simulink subsystem "Vehicle_Model_Simplified"  (R2023b)
settings: Solver=VariableStepAuto  StartTime=0.0  StopTime=10.0  RelTol=1e-3
undefined symbols (not defined in the file): chassis, dZ, F0z, fractalcoef, IMU_accel, IMU_gyro, IMU_mag, phi, powertrain, psi, sim, suspension, theta, VEH, X, Xdot, Y, Ydot, Z, Zdot
libraries: vehdynlibtire x10, vehdynlibsuspension x8, autolibutils x5, sharedtransform x5, shared6dof x2, sensorgpslib x1, mspsensorlib x1, dspstat3 x1, vehdynlibeom x1, vehdynlibtirecommon x1
(part 1 of 6)
settings Model: Creator=Inver  LastModifiedBy=Inver
settings OptimizationCC: ReuseModelBlockBuffer=off

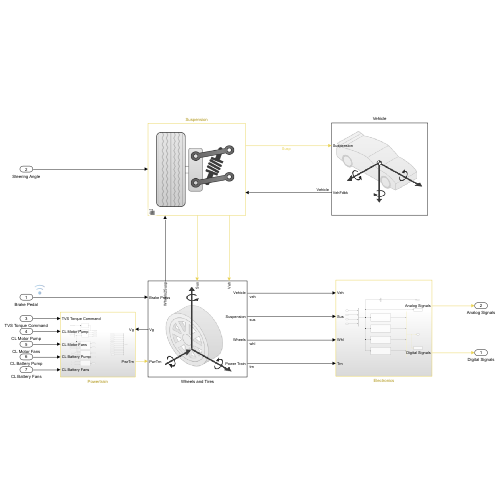
[thumbnail: Simulink's stored preview of the top-level diagram]
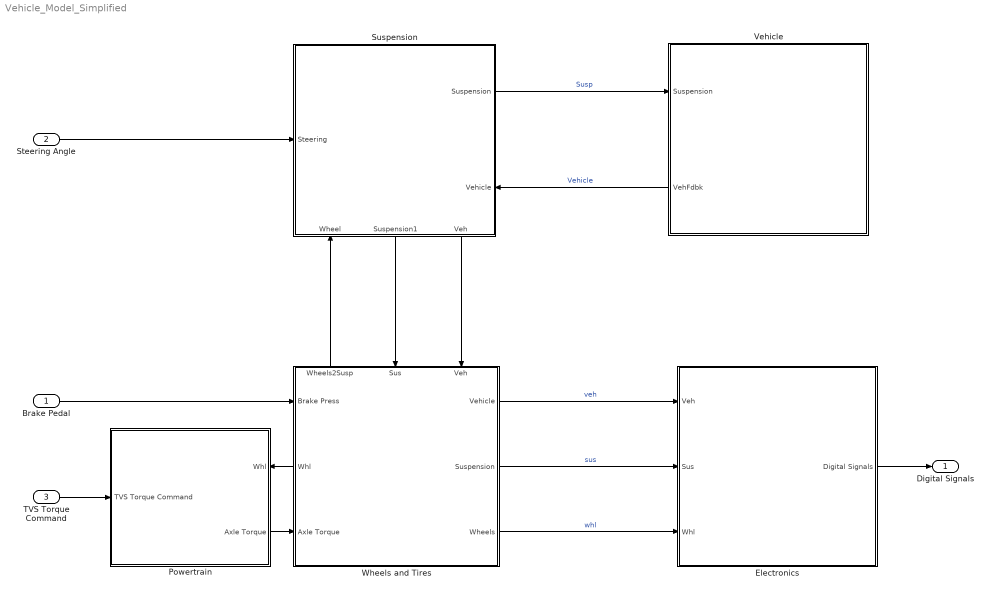
== system Vehicle_Model_Simplified ==
  Brake Pedal : Inport
  Steering Angle : Inport  Port=2
  TVS Torque Command : Inport  Port=3
  Electronics : Subsystem
  Powertrain : Subsystem
      settings: PortSchema="{\"entries\":[{\"content\":{\"sides\":[{\"content\":{\"connectorIds\":[\"In1\"]},\"type\":\"ConnectorPlacement.EquallySpacedRectSide\",\"uuid\":\"0d21e996-4b5b-4450-af88-3d06a2954fb0\"},{\"content\":{\"connectorIds\":[\"In2\",\"Out1\"],\"side\":\"RIGHT\"},\"type\":\"ConnectorPlacement.EquallySpacedRectSide\",\"uuid\":\"9f5ebd0c-1dcb-4dff-b45c-eedc8c3fdf23\"},{\"content\":{\"side\":\"TOP\"},\"type\":\"ConnectorPlacement.EquallySpacedRectSide\",\"uuid\":\"a4defc37-f0d5-4878-ad0c-0744c40eb739\"}]},\"type\":\"ConnectorPlacement.EquallySpacedConnector\",\"uuid\":\"e0fe36d7-0668-4ee0-8075-231a8c6bd792\"}],\"packageUris\":[\"http://schema.mathworks.com/mf0/Connector/R2020b\"],\"version\":\"1.0\"}"
  Suspension : Subsystem  Variant=on  VariantControlMode=label  LabelModeActiveChoice=1
      settings: PortSchema="{\"entries\":[{\"content\":{\"sides\":[{\"content\":{\"connectorIds\":[\"In1\"]},\"type\":\"ConnectorPlacement.EquallySpacedRectSide\",\"uuid\":\"d90bf910-501d-4dd1-a367-d76bd42ab174\"},{\"content\":{\"connectorIds\":[\"Out1\",\"In3\"],\"side\":\"RIGHT\"},\"type\":\"ConnectorPlacement.EquallySpacedRectSide\",\"uuid\":\"1fe7da07-1086-4d5e-8baf-d5d069455d6e\"},{\"content\":{\"connectorIds\":[],\"side\":\"TOP\"},\"type\":\"ConnectorPlacement.EquallySpacedRectSide\",\"uuid\":\"6ff63b9e-45bb-47e9-90cd-47f8e0815e57\"},{\"content\":{\"connectorIds\":[\"In2\",\"Out2\",\"Out3\"],\"side\":\"BOTTOM\"},\"type\":\"ConnectorPlacement.EquallySpacedRectSide\",\"uuid\":\"116c6de0-7bfa-4dc1-bfd0-57a2fffb3aa0\"}]},\"type\":\"ConnectorPlacement.EquallySpacedConnector\",\"uuid\":\"6475b998-12b0-4b0e-8a20-c379b8e08c7c\"}],\"packageUris\":[\"http://schema.mathworks.com/mf0/Connector/R2020b\"],\"version\":\"1.0\"}"
      mask Display:
      | switch str2num(get_param(gcb,'ActiveVariant'))
      |     case 1
      |         image('suspdw.png');
      |     case 2
      |         image([imread('suspindmap.png');imread('suspsamap.png')]);
      |     case 3
      |          image([imread('suspmacp.png');imread('suspsacoil.png')]);
      |     case 4
      |          image('suspmacp.png');
      |     case 5
      |          image('suspindmap.png');
      |     case 6
      |          image('suspkandc.png');
      | end
  Vehicle : Subsystem
      settings: PortSchema="{\"entries\":[{\"content\":{\"sides\":[{\"content\":{\"connectorIds\":[\"In1\",\"Out1\"]},\"type\":\"ConnectorPlacement.EquallySpacedRectSide\",\"uuid\":\"63fa377f-0583-4c60-bac7-9bd73dadd9a1\"},{\"content\":{\"connectorIds\":[],\"side\":\"RIGHT\"},\"type\":\"ConnectorPlacement.EquallySpacedRectSide\",\"uuid\":\"7f668e34-aa5e-4f2f-9be8-80fbb83ff2c8\"},{\"content\":{\"connectorIds\":[],\"side\":\"TOP\"},\"type\":\"ConnectorPlacement.EquallySpacedRectSide\",\"uuid\":\"511f439c-568f-45f1-9ff4-54e644eb8180\"}]},\"type\":\"ConnectorPlacement.EquallySpacedConnector\",\"uuid\":\"b54bf87e-fa06-468b-8fa9-38148d60ed3d\"}],\"packageUris\":[\"http://schema.mathworks.com/mf0/Connector/R2020b\"],\"version\":\"1.0\"}"
      mask Display: image('6dofcar.png');
  Wheels and Tires : Subsystem
      settings: PortSchema="{\"entries\":[{\"content\":{\"sides\":[{\"content\":{\"connectorIds\":[\"In1\",\"Out5\",\"In2\"]},\"type\":\"ConnectorPlacement.EquallySpacedRectSide\",\"uuid\":\"77263124-783e-4307-b979-a6212540af24\"},{\"content\":{\"connectorIds\":[\"Out1\",\"Out2\",\"Out3\"],\"side\":\"RIGHT\"},\"type\":\"ConnectorPlacement.EquallySpacedRectSide\",\"uuid\":\"cb03b446-69c2-4dbf-929b-d33818acfe8b\"},{\"content\":{\"connectorIds\":[\"Out4\",\"In3\",\"In4\"],\"side\":\"TOP\"},\"type\":\"ConnectorPlacement.EquallySpacedRectSide\",\"uuid\":\"8e7e4023-62e5-48a8-8666-b4c8bb14cd01\"}]},\"type\":\"ConnectorPlacement.EquallySpacedConnector\",\"uuid\":\"1061f0db-ec8e-49bd-8d66-b4a53eaeacfa\"}],\"packageUris\":[\"http://schema.mathworks.com/mf0/Connector/R2020b\"],\"version\":\"1.0\"}"
      mask Display: image('wheel3dof.png')
  Digital Signals : Outport  PortDimensions={292}
  wires:
  Wheels and Tires/1(Vehicle) -> Electronics/1(Veh)  "veh"
  Electronics/1(Digital Signals) -> Digital Signals/1
  Vehicle/1(VehFdbk) -> Suspension/3(Vehicle)  "Vehicle"
  Suspension/2(Suspension1) -> Wheels and Tires/3(Sus)
  TVS Torque Command/1 -> Powertrain/1(TVS Torque Command)
  Steering Angle/1 -> Suspension/1(Steering)
  Wheels and Tires/4(Wheels2Susp) -> Suspension/2(Wheel)
  Brake Pedal/1 -> Wheels and Tires/1(Brake Press)
  Wheels and Tires/2(Suspension) -> Electronics/2(Sus)  "sus"
  Suspension/1(Suspension) -> Vehicle/1(Suspension)  "Susp"
  Suspension/3(Veh) -> Wheels and Tires/4(Veh)
  Powertrain/1(Axle Torque) -> Wheels and Tires/2(Axle Torque)
  Wheels and Tires/3(Wheels) -> Electronics/3(Whl)  "whl"
  Wheels and Tires/5(Whl) -> Powertrain/2(Whl)

== system Vehicle_Model_Simplified/Electronics ==
  Veh : Inport
  Sus : Inport  Port=2
  Whl : Inport  Port=3
  All Veh Info : BusCreator  Inputs=3
  Corner Dynamics Sensors : Subsystem
  Digital SIgnals : BusCreator  Inputs=2
  Navigation Sensors : Subsystem
  To Workspace : ToWorkspace  VariableName=Digital_Signals  SaveFormat=Timeseries  SampleTime=-1
  To Workspace1 : ToWorkspace  VariableName=Vehicle_Signals  SaveFormat=Timeseries  SampleTime=-1
  Digital Signals : Outport
  wires:
  Sus/1 -> All Veh Info/2
  Whl/1 -> All Veh Info/3
  Navigation Sensors/1(Navigation Sensors) -> Digital SIgnals/1  "Navigation Sensors"
  Corner Dynamics Sensors/1(Corner Dynamics Sensors) -> Digital SIgnals/2  "Corner Dynamics Sensors"
  Digital SIgnals/1 -> Digital Signals/1, To Workspace/1  "Digital Signls"
  All Veh Info/1 -> To Workspace1/1, Navigation Sensors/1(Analog Signals), Corner Dynamics Sensors/1(Analog Signals)
  Veh/1 -> All Veh Info/1  "veh"

== system Vehicle_Model_Simplified/Powertrain ==
  TVS Torque Command : Inport
  Whl : Inport  Port=2
  Bus Selector : BusSelector  OutputSignals=TireFrame.Omega
  Drivetrain : Subsystem
  Gain : Gain  Gain=sim.top_parameters.MOTOR_ENABLE
  Gain1 : Gain  Gain=powertrain.gearbox.gr
  HV Battery : Subsystem
  Axle Torque : Outport
  wires:
  Gain1/1 -> Drivetrain/3(motor speed)
  Whl/1 -> Bus Selector/1
  Drivetrain/3(wheel torque) -> Axle Torque/1
  Bus Selector/1 -> Gain1/1  "<Omega>"
  TVS Torque Command/1 -> Drivetrain/2(throttle)
  HV Battery/1(battery_V) -> [BattV], Gain/1, Drivetrain/1(battery voltage)
  Drivetrain/1(battery current) -> [BattI], HV Battery/1(battery_I)
  Drivetrain/2(motor current) -> [MotI]
  Gain/1 -> [MotV]

== system Vehicle_Model_Simplified/Suspension ==
  Steering : Inport
  Wheel : Inport  Port=2
  Vehicle : Inport  Port=3
  Double Wishbone Suspension : Subsystem  VariantControl=1
      mask Display: image('suspdw.png');
  Independent Mapped Front Suspension Mapped Solid Axle Rear Suspension : Subsystem  VariantControl=2
      mask Display: image([imread('suspindmap.png');imread('suspsamap.png')]);
  Kinematics and Compliance Independent Suspension : Subsystem  VariantControl=6
      mask Display: image('suspkandc.png');
  MacPherson Front Suspension Solid Axle Rear Suspension : Subsystem  VariantControl=3
      mask Display: image([imread('suspmacp.png');imread('suspsacoil.png')]);
  MacPherson Suspension : Subsystem  VariantControl=4
      mask Display: image('suspmacp.png');
  Mapped Suspension : Subsystem  VariantControl=5
      mask Display: image('suspindmap.png');
  Suspension : Outport  VectorParamsAs1DForOutWhenUnconnected=off
  Suspension1 : Outport  Port=2  VectorParamsAs1DForOutWhenUnconnected=off
  Veh : Outport  Port=3  VectorParamsAs1DForOutWhenUnconnected=off

== system Vehicle_Model_Simplified/Vehicle ==
  Suspension : Inport
  6DOF : Subsystem  VariantControl=1
  Constant : Constant  Value=[0 0 0]
  VehFdbk : Outport  VectorParamsAs1DForOutWhenUnconnected=off
  wires:
  6DOF/1(VehFdbk) -> VehFdbk/1  "VehFdbk"
  Constant/1 -> 6DOF/2(Wind)
  Suspension/1 -> 6DOF/1(Suspension)

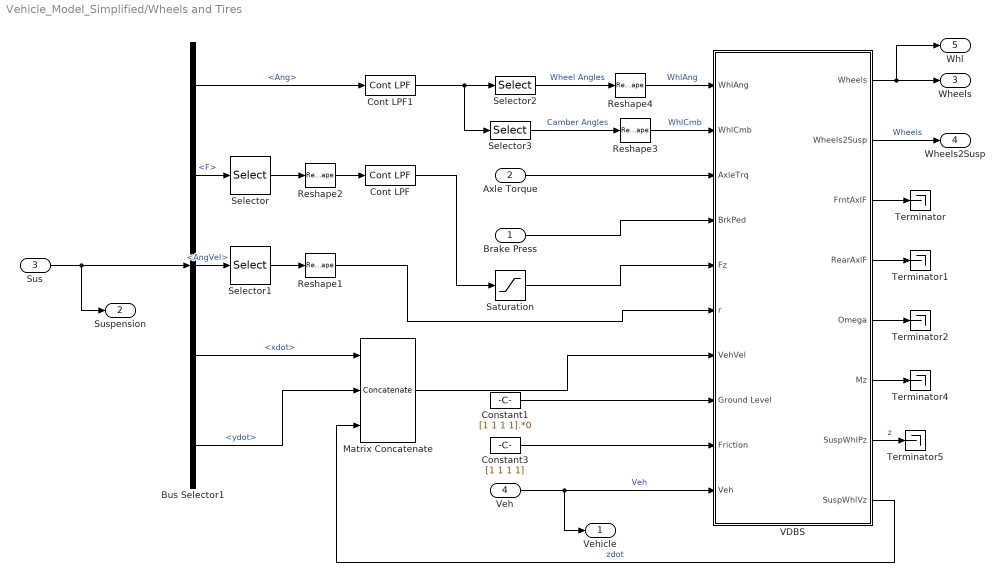
== system Vehicle_Model_Simplified/Wheels and Tires ==
  Brake Press : Inport  Unit=Pa
  Axle Torque : Inport  Port=2
  Sus : Inport  Port=3
  Veh : Inport  Port=4
  Bus Selector1 : BusSelector  OutputSignals=Whl.Ang,Whl.F,Whl.AngVel,Whl.xdot,Whl.ydot
  Constant1 : Constant  Value=[1 1 1 1].*0
  Constant3 : Constant  Value=[1 1 1 1]
  Cont LPF : autolibutils/Cont LPF  wc=100*2*pi  AbsoluteTolerance=auto  aMode=2
  Cont LPF1 : autolibutils/Cont LPF  wc=100*2*pi  AbsoluteTolerance=auto  aMode=2
  Matrix Concatenate : Concatenate  NumInputs=3  Mode=Multidimensional array
  Reshape{1..4} (4 alike) : Reshape
  Saturation : Saturate  UpperLimit=inf  LowerLimit=-10*9.81*2000  ZeroCross=off
  Selector : Selector  NumberOfDimensions=2  InputPortWidth=3  IndexOptions=Index vector (dialog),Select all  Indices=[3],1  OutputSizes=1,1
  Selector1 : Selector  NumberOfDimensions=2  InputPortWidth=1  IndexOptions=Index vector (dialog),Select all  Indices=[3],1  OutputSizes=1,1
  Selector2 : Selector  NumberOfDimensions=2  InputPortWidth=3  IndexOptions=Index vector (dialog),Select all  Indices=3,1  OutputSizes=1,1
  Selector3 : Selector  NumberOfDimensions=2  InputPortWidth=3  IndexOptions=Index vector (dialog),Select all  Indices=1,1  OutputSizes=1,1
  Terminator{,1..2,4..5} (5 alike) : Terminator
  VDBS : Subsystem  VariantControl=0
  Vehicle : Outport  VectorParamsAs1DForOutWhenUnconnected=off
  Suspension : Outport  Port=2  VectorParamsAs1DForOutWhenUnconnected=off
  Wheels : Outport  Port=3  VectorParamsAs1DForOutWhenUnconnected=off
  Wheels2Susp : Outport  Port=4  VectorParamsAs1DForOutWhenUnconnected=off
  Whl : Outport  Port=5  VectorParamsAs1DForOutWhenUnconnected=off
  wires:
  Axle Torque/1 -> VDBS/3(AxleTrq)
  Bus Selector1/2 -> Selector/1  "<F>"
  VDBS/3(FrntAxlF) -> Terminator/1
  VDBS/4(RearAxlF) -> Terminator1/1
  VDBS/6(Mz) -> Terminator4/1
  Selector1/1 -> Reshape1/1
  Matrix Concatenate/1 -> VDBS/7(VehVel)
  Reshape4/1 -> VDBS/1(WhlAng)  "WhlAng"
  Reshape3/1 -> VDBS/2(WhlCmb)  "WhlCmb"
  Selector/1 -> Reshape2/1
  Saturation/1 -> VDBS/5(Fz)
  Constant1/1 -> VDBS/8(Ground Level)
  VDBS/8(SuspWhlVz) -> Matrix Concatenate/3  "zdot"
  Bus Selector1/1 -> Cont LPF1/1  "<Ang>"
  Selector3/1 -> Reshape3/1  "Camber Angles"
  Sus/1 -> Suspension/1, Bus Selector1/1
  Bus Selector1/4 -> Matrix Concatenate/1  "<xdot>"
  Bus Selector1/5 -> Matrix Concatenate/2  "<ydot>"
  VDBS/7(SuspWhlPz) -> Terminator5/1  "z"
  Reshape2/1 -> Cont LPF/1
  Bus Selector1/3 -> Selector1/1  "<AngVel>"
  Reshape1/1 -> VDBS/6(r)
  Brake Press/1 -> VDBS/4(BrkPed)
  Constant3/1 -> VDBS/9(Friction)
  Cont LPF/1 -> Saturation/1
  Cont LPF1/1 -> Selector3/1, Selector2/1
  Selector2/1 -> Reshape4/1  "Wheel Angles"
  Veh/1 -> Vehicle/1, VDBS/10(Veh)  "Veh"
  VDBS/2(Wheels2Susp) -> Wheels2Susp/1  "Wheels"
  VDBS/1(Wheels) -> Wheels/1, Whl/1
  VDBS/5(Omega) -> Terminator2/1

== system Vehicle_Model_Simplified/Electronics/Corner Dynamics Sensors ==
  Analog Signals : Inport
  Bus Creator10 : BusCreator  Inputs=4
  Bus Selector : BusSelector  OutputSignals=whl.TireFrame.Omega,sus.Sus.steering_angle,sus.Sus.shock_length,whl.TireFrame.GndFz
  Delay15 : Delay  InitialCondition=ones(1, 4, 2).*sim.IC.omega_IC
  Delay16 : Delay  InitialCondition=[1 1].*sim.IC.theta_IC
  Delay17 : Delay  InitialCondition=[1 1; 1 1; 1 1; 1 1].*sim.IC.shock_length_IC
  Delay18 : Delay  InitialCondition=[1 1; 1 1; 1 1; 1 1].*sim.IC.Fz_IC
  Saturation15 : Saturate  UpperLimit=sim.range.SHOCK_LENGTH_MAX  LowerLimit=sim.range.SHOCK_LENGTH_MIN
  Saturation16 : Saturate  UpperLimit=sim.range.OMEGA_MAX  LowerLimit=sim.range.OMEGA_MIN
  Saturation17 : Saturate  UpperLimit=sim.range.FZ_MAX  LowerLimit=sim.range.FZ_MIN
  Saturation3 : Saturate  UpperLimit=sim.range.CENTER_STEER_ANGLE_MAX  LowerLimit=-sim.range.CENTER_STEER_ANGLE_MAX
  Transpose : Math  Operator=transpose
  Zero-Order Hold{15..18} (4 alike) : ZeroOrderHold  SampleTime=sim.timing.duplicate
  Corner Dynamics Sensors : Outport
  wires:
  Transpose/1 -> Zero-Order Hold15/1  "omega"
  Bus Selector/1 -> Transpose/1  "<Omega>"
  Zero-Order Hold18/1 -> Delay18/1
  Delay18/1 -> Saturation17/1
  Zero-Order Hold15/1 -> Delay15/1
  Zero-Order Hold16/1 -> Delay16/1
  Saturation17/1 -> Bus Creator10/4  "FZ"
  Saturation3/1 -> Bus Creator10/2  "theta"
  Bus Selector/3 -> Zero-Order Hold17/1  "<shock_length>"
  Saturation15/1 -> Bus Creator10/3  "shock_L"
  Saturation16/1 -> Bus Creator10/1  "omega"
  Bus Selector/4 -> Zero-Order Hold18/1  "<GndFz>"
  Delay16/1 -> Saturation3/1
  Bus Selector/2 -> Zero-Order Hold16/1  "<steering_angle>"
  Delay17/1 -> Saturation15/1
  Delay15/1 -> Saturation16/1
  Zero-Order Hold17/1 -> Delay17/1
  Bus Creator10/1 -> Corner Dynamics Sensors/1
  Analog Signals/1 -> Bus Selector/1

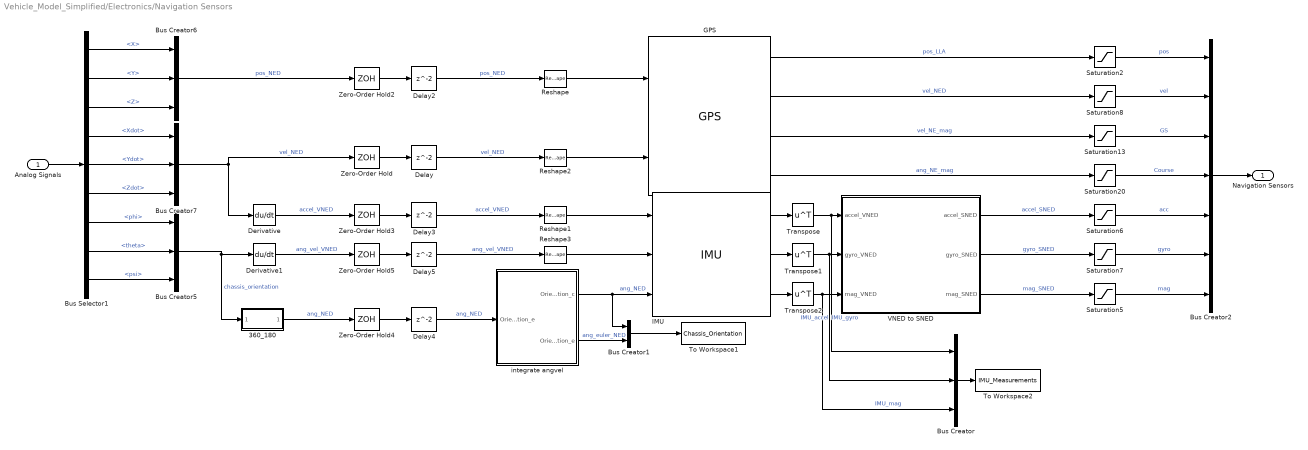
== system Vehicle_Model_Simplified/Electronics/Navigation Sensors ==
  Analog Signals : Inport
  360_180 : Subsystem
  Bus Creator : BusCreator  Inputs=IMU_accel,IMU_gyro,IMU_mag
  Bus Creator1 : BusCreator  Inputs=2
  Bus Creator2 : BusCreator  Inputs=7
  Bus Creator5 : BusCreator  Inputs=phi,theta,psi
  Bus Creator6 : BusCreator  Inputs=X,Y,Z
  Bus Creator7 : BusCreator  Inputs=Xdot,Ydot,Zdot
  Bus Selector1 : BusSelector  OutputSignals=veh.InertFrm.Cg.Disp.X,veh.InertFrm.Cg.Disp.Y,veh.InertFrm.Cg.Disp.Z,veh.InertFrm.Cg.Vel.Xdot,veh.InertFrm.Cg.Vel.Ydot,veh.InertFrm.Cg.Vel.Zdot,veh.InertFrm.Cg.Ang.phi,veh.InertFrm.Cg.Ang.theta,veh.InertFrm.Cg.Ang.psi
  Delay : Delay  InitialCondition=([1;1]*sim.IC.vel_IC)'
  Delay2 : Delay  InitialCondition=[1 1; 1 1; 1 1].*sim.IC.pos_IC
  Delay3 : Delay  InitialCondition=[1 1; 1 1; 1 1].*sim.IC.acc_IC
  Delay4 : Delay  InitialCondition=[1 1; 1 1; 1 1].*sim.IC.ang_IC
  Delay5 : Delay  InitialCondition=[1 1; 1 1; 1 1].*sim.IC.ang_vel_IC
  Derivative : Derivative
  Derivative1 : Derivative
  GPS : sensorgpslib/GPS  DispRefFrame=NED  PositionInputFormat=Local  ReferenceLocation=sim.IC.location_lla_IC  HorizontalPositionAccuracy=sensor.gps.GPS_Z_ACCURACY  VerticalPositionAccuracy=sensor.gps.GPS_XY_ACCURACY  VelocityAccuracy=sensor.gps.GPS_V_ACCURACY  DecayFactor=sensor.gps.GPS_NOISE_FACTOR  SeedDouble=sensor.gps.r_GPS  SimulateUsing=Interpreted execution
      settings: LibrarySourceBlock=mspsensorlib/GPS
  IMU : mspsensorlib/IMU  DispRefFrame=NED  TemperaturePort=off  Temperature=25  MagneticFieldPort=off  MagneticFieldNED=sim.IC.mag_field_IC  MagneticFieldENU=[ -2.4169, 27.5550, 16.0849 ]  SeedDouble=sensor.imu.r_IMU  SimulateUsing=Interpreted execution  AccelParamsMeasurementRange=sensor.imu.ACC_MAX  AccelParamsResolution=sensor.imu.ACC_RES  AccelParamsConstantBias=sensor.imu.ACC_BIAS  AccelParamsAxesMisalignment=sensor.imu.ACC_SKEW  AccelParamsNoiseDensity=sensor.imu.ACC_VEL_WALK  AccelParamsBiasInstability=sensor.imu.ACC_BIAS_INSTABILITY  AccelParamsBiasInstabilityNumerator=fractalcoef().Numerator  AccelParamsBiasInstabilityDenominator=fractalcoef().Denominator  AccelParamsRandomWalk=sensor.imu.ACC_WALK  AccelParamsNoiseType=double-sided  AccelParamsTemperatureBias=sensor.imu.ACC_T_BIAS  AccelParamsTemperatureScaleFactor=sensor.imu.ACC_T_SCALE  GyroParamsMeasurementRange=sensor.imu.GYR_MAX  GyroParamsResolution=sensor.imu.GYR_RES  GyroParamsConstantBias=sensor.imu.GYR_BIAS  GyroParamsAxesMisalignment=sensor.imu.GYR_SKEW  GyroParamsAccelerationBias=sensor.imu.GYR_ACC_BIAS  GyroParamsNoiseDensity=sensor.imu.GYR_ANG_WALK  GyroParamsBiasInstability=sensor.imu.GYR_BIAS_INSTABILITY  GyroParamsBiasInstabilityNumerator=fractalcoef().Numerator  GyroParamsBiasInstabilityDenominator=fractalcoef().Denominator  GyroParamsRandomWalk=sensor.imu.GYR_WALK  GyroParamsNoiseType=double-sided  GyroParamsTemperatureBias=sensor.imu.GYR_T_BIAS  GyroParamsTemperatureScaleFactor=sensor.imu.GYR_T_SCALE  MagParamsMeasurementRange=sensor.imu.MAG_MAX  MagParamsResolution=sensor.imu.MAG_RES  MagParamsConstantBias=sensor.imu.MAG_BIAS  MagParamsAxesMisalignment=sensor.imu.MAG_SKEW  MagParamsNoiseDensity=sensor.imu.MAG_WHITE  MagParamsBiasInstability=sensor.imu.MAG_BIAS_INSTABILITY  MagParamsBiasInstabilityNumerator=fractalcoef().Numerator  MagParamsBiasInstabilityDenominator=fractalcoef().Denominator  MagParamsRandomWalk=sensor.imu.MAG_WALK  MagParamsNoiseType=double-sided  MagParamsTemperatureBias=sensor.imu.MAG_T_BIAS  MagParamsTemperatureScaleFactor=sensor.imu.MAG_T_SCALE
  Reshape{,1..3} (4 alike) : Reshape  OutputDimensionality=Row vector (2-D)
  Saturation13 : Saturate  UpperLimit=sim.range.VELOCITY_MAX  LowerLimit=-sim.range.VELOCITY_MAX
  Saturation2 : Saturate  UpperLimit=inf  LowerLimit=-inf
  Saturation20 : Saturate  UpperLimit=sim.range.ORIENTATION_MAX  LowerLimit=-sim.range.ORIENTATION_MAX
  Saturation5 : Saturate  UpperLimit=sim.range.MAG_MAX  LowerLimit=-sim.range.MAG_MAX
  Saturation6 : Saturate  UpperLimit=sim.range.ACCELERATION_MAX  LowerLimit=-sim.range.ACCELERATION_MAX
  Saturation7 : Saturate  UpperLimit=sim.range.YAW_MAX  LowerLimit=-sim.range.YAW_MAX
  Saturation8 : Saturate  UpperLimit=sim.range.VELOCITY_MAX  LowerLimit=-sim.range.VELOCITY_MAX
  To Workspace1 : ToWorkspace  VariableName=Chassis_Orientation  SaveFormat=Timeseries  SampleTime=-1
  To Workspace2 : ToWorkspace  VariableName=IMU_Measurements  SaveFormat=Timeseries  SampleTime=-1
  Transpose : Math  Operator=transpose
  Transpose1 : Math  Operator=transpose
  Transpose2 : Math  Operator=transpose
  VNED to SNED : MATLAB Function  TreatAsAtomicUnit=on
  Zero-Order Hold{,2..5} (5 alike) : ZeroOrderHold  SampleTime=sim.timing.duplicate
  integrate angvel : MATLAB Function  TreatAsAtomicUnit=on
  Navigation Sensors : Outport
  wires:
  Delay5/1 -> Reshape3/1  "ang_vel_VNED"
  Delay/1 -> Reshape2/1  "vel_NED"
  Delay3/1 -> Reshape1/1  "accel_VNED"
  Delay2/1 -> Reshape/1  "pos_NED"
  integrate angvel/1(Orientation_c) -> Bus Creator1/1, IMU/3  "ang_NED"
  GPS/4 -> Saturation20/1  "ang_NE_mag"
  GPS/3 -> Saturation13/1  "vel_NE_mag"
  GPS/2 -> Saturation8/1  "vel_NED"
  GPS/1 -> Saturation2/1  "pos_LLA"
  VNED to SNED/2(gyro_SNED) -> Saturation7/1  "gyro_SNED"
  VNED to SNED/1(accel_SNED) -> Saturation6/1  "accel_SNED"
  VNED to SNED/3(mag_SNED) -> Saturation5/1  "mag_SNED"
  Delay4/1 -> integrate angvel/1("Orientation_e ")  "ang_NED"
  Transpose2/1 -> Bus Creator/3, VNED to SNED/3(mag_VNED)  "IMU_mag"
  Transpose1/1 -> Bus Creator/2, VNED to SNED/2(gyro_VNED)  "IMU_gyro"
  Transpose/1 -> Bus Creator/1, VNED to SNED/1(accel_VNED)  "IMU_accel"
  IMU/3 -> Transpose2/1
  IMU/1 -> Transpose/1
  IMU/2 -> Transpose1/1
  Bus Creator/1 -> To Workspace2/1
  Bus Creator1/1 -> To Workspace1/1
  integrate angvel/2(Orientation_e) -> Bus Creator1/2  "ang_euler_NED"
  Zero-Order Hold/1 -> Delay/1
  Bus Creator7/1 -> Zero-Order Hold/1, Derivative/1  "vel_NED"
  Zero-Order Hold2/1 -> Delay2/1
  Bus Creator6/1 -> Zero-Order Hold2/1  "pos_NED"
  Zero-Order Hold3/1 -> Delay3/1
  Derivative/1 -> Zero-Order Hold3/1  "accel_VNED"
  Zero-Order Hold5/1 -> Delay5/1
  Derivative1/1 -> Zero-Order Hold5/1  "ang_vel_VNED"
  Zero-Order Hold4/1 -> Delay4/1
  360_180/1(psi_rev) -> Zero-Order Hold4/1  "ang_NED"
  Saturation2/1 -> Bus Creator2/1  "pos"
  Saturation13/1 -> Bus Creator2/3  "GS"
  Saturation6/1 -> Bus Creator2/5  "acc"
  Saturation20/1 -> Bus Creator2/4  "Course"
  Saturation5/1 -> Bus Creator2/7  "mag"
  Saturation8/1 -> Bus Creator2/2  "vel"
  Saturation7/1 -> Bus Creator2/6  "gyro"
  Bus Creator2/1 -> Navigation Sensors/1
  Bus Selector1/1 -> Bus Creator6/1  "<X>"
  Bus Selector1/8 -> Bus Creator5/2  "<theta>"
  Bus Selector1/2 -> Bus Creator6/2  "<Y>"
  Bus Selector1/6 -> Bus Creator7/3  "<Zdot>"
  Bus Selector1/5 -> Bus Creator7/2  "<Ydot>"
  Bus Selector1/4 -> Bus Creator7/1  "<Xdot>"
  Bus Selector1/7 -> Bus Creator5/1  "<phi>"
  Bus Creator5/1 -> 360_180/1(<psi>), Derivative1/1  "chassis_orientation"
  Bus Selector1/3 -> Bus Creator6/3  "<Z>"
  Bus Selector1/9 -> Bus Creator5/3  "<psi>"
  Analog Signals/1 -> Bus Selector1/1
  Reshape/1 -> GPS/1
  Reshape1/1 -> IMU/1
  Reshape2/1 -> GPS/2
  Reshape3/1 -> IMU/2

== system Vehicle_Model_Simplified/Powertrain/Drivetrain ==
  battery voltage : Inport
  throttle : Inport  Port=2
  motor speed : Inport  Port=3
  1-D Lookup Table : Lookup_n-D  NumberOfTableDimensions=1  LookupTableObject=''  BreakpointsForDimension1=powertrain.motor.speed_bp  BreakpointsForDimension1FirstPoint=10  BreakpointsForDimension2FirstPoint=10  BreakpointsForDimension1Spacing=12  BreakpointsForDimension2Spacing=12  BeginIndexSearchUsingPreviousIndexResult=on  Table=powertrain.motor.max_torque_table  ExtrapMethod=Clip  DiagnosticForOutOfRangeInput=Error  InternalRulePriority=Speed  RndMeth=Simplest
  1-D Lookup Table1 : Lookup_n-D  NumberOfTableDimensions=1  LookupTableObject=''  BreakpointsForDimension1=powertrain.motor.speed_bp  BreakpointsForDimension1FirstPoint=10  BreakpointsForDimension2FirstPoint=10  BreakpointsForDimension1Spacing=12  BreakpointsForDimension2Spacing=12  BeginIndexSearchUsingPreviousIndexResult=on  Table=powertrain.motor.max_current_table  ExtrapMethod=Clip  DiagnosticForOutOfRangeInput=Error  InternalRulePriority=Speed  RndMeth=Simplest
  Gain : Gain  Gain=sim.top_parameters.MOTOR_ENABLE
  Gain1 : Gain  Gain=powertrain.gearbox.gr.*powertrain.gearbox.ge
  Gain2 : Gain  Gain=sim.top_parameters.MOTOR_ENABLE
  Mean : dspstat3/Mean  run=off  InputProcessing=Columns as channels (frame based)  reset_popup=None  directionMode=Entire input  dimension=1  roiEnable=off  roiType=Rectangles  roiPortion=Entire ROI  roiOutput=Individual statistics for each ROI  roiFlag=off  roundingMode=Floor  overflowMode=off  outputDataTypeStr=Inherit: Same as accumulator  outputMin=[]  outputMax=[]  outputLastDataTypeStr=Inherit: Same as accumulator
  Product : Product
  Product1 : Product
  Sum : Sum  Inputs=+
  Terminator : Terminator
  battery current : Outport
  motor current : Outport  Port=2
  wheel torque : Outport  Port=3
  wires:
  1-D Lookup Table/1 -> Gain/1
  motor speed/1 -> 1-D Lookup Table1/1, Mean/1
  Product/1 -> Gain1/1
  throttle/1 -> Product/1, Product1/1
  Gain/1 -> Product/2
  Gain1/1 -> wheel torque/1
  Sum/1 -> battery current/1
  battery voltage/1 -> Terminator/1
  Mean/1 -> 1-D Lookup Table/1
  1-D Lookup Table1/1 -> Gain2/1
  Gain2/1 -> Product1/2
  Product1/1 -> motor current/1, Sum/1

== system Vehicle_Model_Simplified/Powertrain/HV Battery ==
  battery_I : Inport
  1-D Lookup Table : Lookup_n-D  NumberOfTableDimensions=1  BreakpointsForDimension1=powertrain.battery.SOC  Table=powertrain.battery.Em  InternalRulePriority=Speed  RndMeth=Simplest
  Constant1 : Constant  Value=sim.IC.SOC_IC
  Gain : Gain  Gain=1/(3600*powertrain.battery.Np*powertrain.battery.Ah)
  Gain1 : Gain  Gain=powertrain.battery.Ns
  Gain2 : Gain  Gain=powertrain.battery.R
  Integrator : Integrator
  Sum1 : Sum  Inputs=|+-
  Sum2 : Sum  Inputs=|+-
  battery_V : Outport
  wires:
  Gain/1 -> Sum1/2
  Constant1/1 -> Sum1/1
  Gain2/1 -> Sum2/2
  Integrator/1 -> Gain/1
  Sum2/1 -> battery_V/1
  battery_I/1 -> Gain2/1, Integrator/1
  Sum1/1 -> 1-D Lookup Table/1  "SOC"
  1-D Lookup Table/1 -> Gain1/1
  Gain1/1 -> Sum2/1

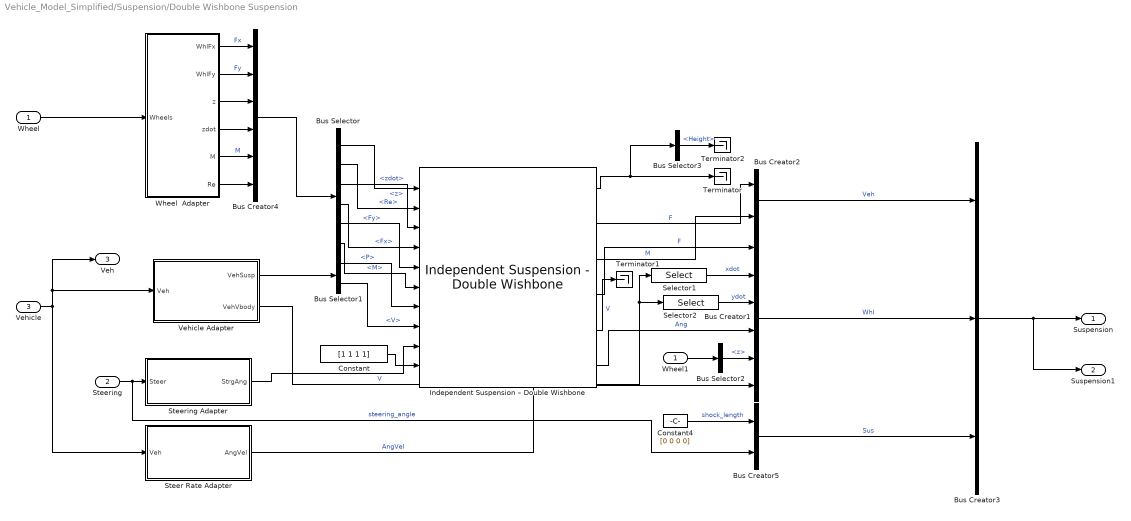
== system Vehicle_Model_Simplified/Suspension/Double Wishbone Suspension ==
  Wheel : Inport
  Steering : Inport  Port=2
  Vehicle : Inport  Port=3
  Bus Creator1 : BusCreator  Inputs=6
  Bus Creator2 : BusCreator  Inputs=2
  Bus Creator3 : BusCreator  Inputs=3
  Bus Creator4 : BusCreator  Inputs=6
  Bus Creator5 : BusCreator  Inputs=2
  Bus Selector : BusSelector  OutputSignals=z,Re,zdot,Fx,Fy,M
  Bus Selector1 : BusSelector  OutputSignals=P,V
  Bus Selector2 : BusSelector  OutputSignals=SuspFrame.z
  Bus Selector3 : BusSelector  OutputSignals=Height
  Constant : Constant  Value=[1 1 1 1]
  Constant4 : Constant  Value=[0 0 0 0]
  Independent Suspension – Double Wishbone : vehdynlibsuspension/Independent Suspension - Double Wishbone  ActiveDampEn=on  NumAxl=2  NumWhlsByAxl=[2 2]  StrgEnByAxl=[1 0]  AntiSwayEnByAxl=[0 1]  WhlNumVec="[1  2  1  2]"  AxleNumVec="[1  1  2  2]"  SuspTypesByAxle="[1  1]"  SuspImage=suspdw.png  IdealSuspEn=on  IdealSuspAxles="[1  2]"  Kz=suspension.shock.Kz  F0z=suspension.shock.F0z  Cz=Cz  Hmax=suspension.shock.Hmax  f_act_susp_cz=suspension.shock.f_act_susp_cz  f_act_susp_duty_bpt=suspension.shock.f_act_susp_duty_bpt  f_act_susp_zdot_bpt=suspension.shock.f_act_susp_zdot_bpt  Toe=0.  RollStrgSlp=0.  ToeStrgSlp=0.  Caster=0.  CasterHslp=0.  CasterStrgSlp=0.  Camber=0.  CamberHslp=0.  CamberStrgSlp=0.  StrgHgtSlp=0.  MappedSuspEn=off  MappedSuspAxles="[1  2]"  f_susp_axl_bp=[1 2]  f_susp_dz_bp=[-0.15 -0.14 -0.13 -0.12 -0.11 -0.10 -0.09 -0.08 -0.07 -0.06 -0.05 -0.04 -0.03 -0.02 -0.01 0.00 0.01 0.02 0.03 0.04 0.05 0.06 0.07 0.08 0.09 0.10 0.11 0.12 0.13 0.14 0.15]  f_susp_dzdot_bp=[-0.15 -0.14 -0.13 -0.12 -0.11 -0.10 -0.09 -0.08 -0.07 -0.06 -0.05 -0.04 -0.03 -0.02 -0.01 0.00 0.01 0.02 0.03 0.04 0.05 0.06 0.07 0.08 0.09 0.10 0.11 0.12 0.13 0.14 0.15]  f_susp_fmz=zeros(31,31,61,2,4)  f_susp_geom=zeros(31,61,2,3)  f_susp_strgdelta_bp=[-30,-29,-28,-27,-26,-25,-24,-23,-22,-21,-20,-19,-18,-17,-16,-15,-14,-13,-12,-11,-10,-9,-8,-7,-6,-5,-4,-3,-2,-1,0,1,2,3,4,5,6,7,8,9,10,11,12,13,14,15,16,17,18,19,20,21,22,23,24,25,26,27,28,29,30]  AntiSwayR=suspension.arb.AntiSwayR  AntiSwayNtrlAng=suspension.arb.AntiSwayNtrlAng  AntiSwayTrsK=suspension.arb.AntiSwayTrsK
  Selector1 : Selector  NumberOfDimensions=2  IndexOptions=Index vector (dialog),Select all  Indices=1,1  OutputSizes=1,1
  Selector2 : Selector  NumberOfDimensions=2  IndexOptions=Index vector (dialog),Select all  Indices=2,1  OutputSizes=1,1
  Steer Rate Adapter : Subsystem
  Steering Adapter : Subsystem
  Terminator : Terminator
  Terminator1 : Terminator
  Terminator2 : Terminator
  Vehicle Adapter : Subsystem
  Wheel  Adapter : Subsystem
  Wheel1 : InportShadow
  Suspension : Outport  VectorParamsAs1DForOutWhenUnconnected=off
  Suspension1 : Outport  Port=2  VectorParamsAs1DForOutWhenUnconnected=off
  Veh : Outport  Port=3  VectorParamsAs1DForOutWhenUnconnected=off
  wires:
  Bus Creator3/1 -> Suspension/1, Suspension1/1
  Steering Adapter/1(StrgAng) -> Independent Suspension – Double Wishbone/9
  Independent Suspension – Double Wishbone/1 -> Bus Selector3/1, Terminator/1
  Wheel  Adapter/6(Re) -> Bus Creator4/6
  Bus Selector1/1 -> Independent Suspension – Double Wishbone/7  "<P>"
  Wheel  Adapter/2(WhlFy) -> Bus Creator4/2  "Fy"
  Wheel/1 -> Wheel  Adapter/1(Wheels)
  Steer Rate Adapter/1(AngVel) -> Bus Creator1/6  "AngVel"
  Bus Creator4/1 -> Bus Selector/1
  Bus Creator2/1 -> Bus Creator3/1  "Veh"
  Vehicle Adapter/2(VehVbody) -> Selector1/1, Selector2/1  "V"
  Selector2/1 -> Bus Creator1/3  "ydot"
  Bus Selector1/2 -> Independent Suspension – Double Wishbone/8  "<V>"
  Independent Suspension – Double Wishbone/2 -> Bus Creator2/1  "F"
  Bus Selector/2 -> Independent Suspension – Double Wishbone/2  "<Re>"
  Wheel  Adapter/5(M) -> Bus Creator4/5  "M"
  Bus Selector/4 -> Independent Suspension – Double Wishbone/4  "<Fx>"
  Independent Suspension – Double Wishbone/4 -> Bus Creator1/1  "F"
  Selector1/1 -> Bus Creator1/2  "xdot"
  Independent Suspension – Double Wishbone/3 -> Bus Creator2/2  "M"
  Vehicle Adapter/1(VehSusp) -> Bus Selector1/1
  Wheel  Adapter/4(zdot) -> Bus Creator4/4
  Vehicle/1 -> Veh/1, Vehicle Adapter/1(Veh), Steer Rate Adapter/1(Veh)
  Bus Selector/6 -> Independent Suspension – Double Wishbone/6  "<M>"
  Bus Selector/5 -> Independent Suspension – Double Wishbone/5  "<Fy>"
  Bus Selector/1 -> Independent Suspension – Double Wishbone/1  "<z>"
  Wheel  Adapter/3(z) -> Bus Creator4/3
  Independent Suspension – Double Wishbone/6 -> Bus Creator1/4  "Ang"
  Bus Creator1/1 -> Bus Creator3/2  "Whl"
  Wheel  Adapter/1(WhlFx) -> Bus Creator4/1  "Fx"
  Bus Selector/3 -> Independent Suspension – Double Wishbone/3  "<zdot>"
  Independent Suspension – Double Wishbone/5 -> Terminator1/1  "V"
  Bus Selector2/1 -> Bus Creator1/5  "<z>"
  Wheel1/1 -> Bus Selector2/1
  Constant4/1 -> Bus Creator5/1  "shock_length"
  Bus Creator5/1 -> Bus Creator3/3  "Sus"
  Steering/1 -> Bus Creator5/2, Steering Adapter/1(Steer)  "steering_angle"
  Bus Selector3/1 -> Terminator2/1  "<Height>"
  Constant/1 -> Independent Suspension – Double Wishbone/10

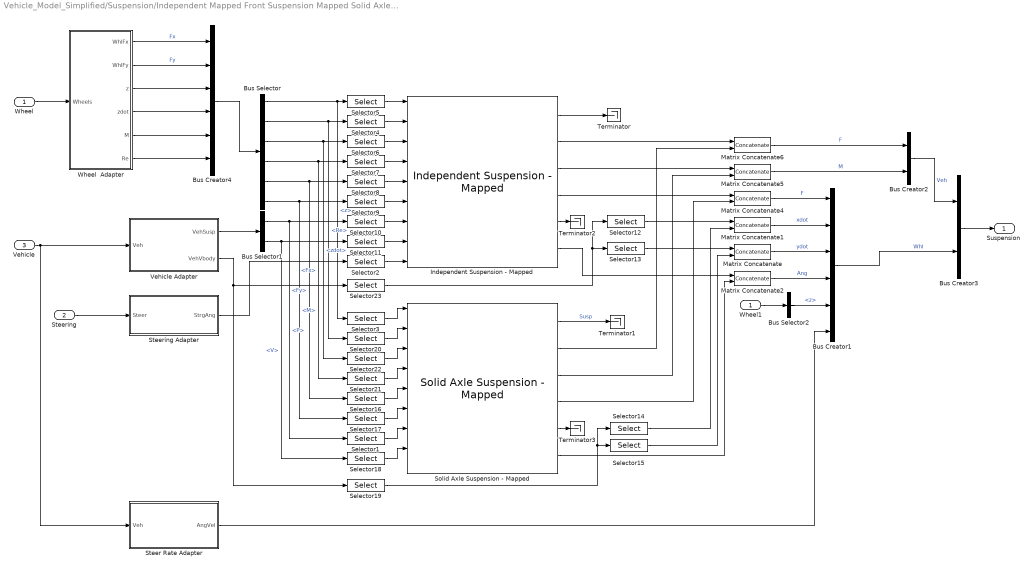
== system Vehicle_Model_Simplified/Suspension/Independent Mapped Front Suspension Mapped Solid Axle Rear Suspension ==
  Wheel : Inport
  Steering : Inport  Port=2
  Vehicle : Inport  Port=3
  Bus Creator1 : BusCreator  Inputs=6
  Bus Creator2 : BusCreator  Inputs=2
  Bus Creator3 : BusCreator  Inputs=2
  Bus Creator4 : BusCreator  Inputs=6
  Bus Selector : BusSelector  OutputSignals=z,Re,zdot,Fx,Fy,M
  Bus Selector1 : BusSelector  OutputSignals=P,V
  Bus Selector2 : BusSelector  OutputSignals=SuspFrame.z
  Independent Suspension - Mapped : vehdynlibsuspension/Independent Suspension - Mapped  NumAxl=1  NumWhlsByAxl=[2 2]  StrgEnByAxl=1  AntiSwayEnByAxl=1  WhlNumVec="[1  2  1  2]"  AxleNumVec="[1  1]"  SuspTypesByAxle=[2]  SuspImage=suspindmap.png  IdealSuspEn=off  IdealSuspAxles="[1  2]"  Kz=64370  F0z=9810  Cz=10000  Hmax=0.5  Toe=2  RollStrgSlp=-13  ToeStrgSlp=0.01  Caster=4  CasterHslp=-13  CasterStrgSlp=0.01  Camber=4  CamberHslp=-13  CamberStrgSlp=0.01  StrgHgtSlp=0.0025  MappedSuspEn=on  MappedSuspAxles=[1]  f_susp_axl_bp=[1 2]  f_susp_dz_bp=f_susp_dz_bp  f_susp_dzdot_bp=f_susp_dzdot_bp  f_susp_fmz=f_susp_fmz  f_susp_geom=f_susp_geom  f_susp_strgdelta_bp=f_susp_strgdelta_bp  NDFLookupOutType=1:4  NDGLookupOutType=1:3  AntiSwayR=0.2  AntiSwayNtrlAng=0.5236  AntiSwayTrsK=8e2
      link override For each track and axle combination calculate suspension forces and moments/Suspension/Suspension Angle Calculations: OverrideUsingVariant=MappedSteeringEnabled
      link override For each track and axle combination calculate suspension forces and moments/Suspension/Z axis suspension characteristic: OverrideUsingVariant=MappedSuspension
  Matrix Concatenate{,1..2,4..6} (6 alike) : Concatenate  Mode=Multidimensional array  ConcatenateDimension=2
  Selector{1,17..19} (4 alike) : Selector  NumberOfDimensions=2  IndexOptions=Select all,Index vector (dialog)  Indices=[1 2],[3 4]  OutputSizes=1,1
  Selector{9..11,23} (4 alike) : Selector  NumberOfDimensions=2  IndexOptions=Select all,Index vector (dialog)  Indices=[1 2],[1 2]  OutputSizes=1,1
  Selector12 : Selector  NumberOfDimensions=2  InputPortWidth=3  IndexOptions=Index vector (dialog),Select all  Indices=1,1  OutputSizes=1,1
  Selector13 : Selector  NumberOfDimensions=2  InputPortWidth=3  IndexOptions=Index vector (dialog),Select all  Indices=2,1  OutputSizes=1,1
  Selector14 : Selector  NumberOfDimensions=2  InputPortWidth=3  IndexOptions=Index vector (dialog),Select all  Indices=1,1  OutputSizes=1,1
  Selector15 : Selector  NumberOfDimensions=2  InputPortWidth=3  IndexOptions=Index vector (dialog),Select all  Indices=2,1  OutputSizes=1,1
  Selector{3,16,20..22} (5 alike) : Selector  IndexOptions=Index vector (dialog)  Indices=[3 4]  OutputSizes=1
  Selector{2,4..8} (6 alike) : Selector  IndexOptions=Index vector (dialog)  Indices=[1 2]  OutputSizes=1
  Solid Axle Suspension - Mapped : vehdynlibsuspension/Solid Axle Suspension - Mapped  NumAxl=1  NumWhlsByAxl=[2 2]  StrgEnByAxl=0  WhlNumVec="[1  2  1  2]"  AxleNumVec="[1  1]"  SuspTypesByAxle=[2]  SuspImage=suspsamap.png  AxlIxx=AxlIxx  AxlM=AxlM  TrackCoords=[0 0;VEH.TrackWidth*[-1 1]/2;0 0]  SuspCoords=[0 0;VEH.TrackWidth*[-1 1]/2;0 0]  KzWhlAxl=KzWhlAxl  F0zWhlAxl=F0zWhlAxl  CzWhlAxl=CzWhlAxl  IdealSuspEn=off  IdealSuspAxles="[1  2]"  Kz=64370  F0z=9810  Cz=10000  Hmax=0.5  Toe=2  RollStrgSlp=-13  ToeStrgSlp=0.01  Caster=4  CasterHslp=-13  CasterStrgSlp=0.01  Camber=4  CamberHslp=-13  CamberStrgSlp=0.01  StrgHgtSlp=0.0025  MappedSuspEn=on  MappedSuspAxles=[1]  f_susp_axl_bp=[1 2]  f_susp_dz_bp=f_susp_dz_bp  f_susp_dzdot_bp=f_susp_dzdot_bp  f_susp_fmz=f_susp_fmz  f_susp_geom=f_susp_geom  f_susp_strgdelta_bp=f_susp_strgdelta_bp  NDFLookupOutType=1:4  NDGLookupOutType=1:3
      link override For each track and axle combination calculate suspension forces and moments/Suspension/Suspension Angle Calculations: OverrideUsingVariant=MappedSteeringEnabled
      link override For each track and axle combination calculate suspension forces and moments/Suspension/Z axis suspension characteristic: OverrideUsingVariant=MappedSuspension
  Steer Rate Adapter : Subsystem
  Steering Adapter : Subsystem
  Terminator{,1..3} (4 alike) : Terminator
  Vehicle Adapter : Subsystem
  Wheel  Adapter : Subsystem
  Wheel1 : InportShadow
  Suspension : Outport  VectorParamsAs1DForOutWhenUnconnected=off
  wires:
  Vehicle Adapter/2(VehVbody) -> Selector19/1, Selector23/1
  Selector22/1 -> Solid Axle Suspension - Mapped/3
  Bus Selector/3 -> Selector22/1, Selector6/1  "<zdot>"
  Solid Axle Suspension - Mapped/4 -> Matrix Concatenate4/2
  Solid Axle Suspension - Mapped/1 -> Terminator1/1  "Susp"
  Selector12/1 -> Matrix Concatenate1/1
  Selector7/1 -> Independent Suspension - Mapped/4
  Selector18/1 -> Solid Axle Suspension - Mapped/8
  Selector13/1 -> Matrix Concatenate/1
  Selector14/1 -> Matrix Concatenate1/2
  Selector21/1 -> Solid Axle Suspension - Mapped/4
  Vehicle/1 -> Vehicle Adapter/1(Veh), Steer Rate Adapter/1(Veh)
  Wheel  Adapter/4(zdot) -> Bus Creator4/4
  Solid Axle Suspension - Mapped/3 -> Matrix Concatenate5/2
  Selector1/1 -> Solid Axle Suspension - Mapped/7
  Matrix Concatenate4/1 -> Bus Creator1/1  "F"
  Selector16/1 -> Solid Axle Suspension - Mapped/5
  Matrix Concatenate5/1 -> Bus Creator2/2  "M"
  Independent Suspension - Mapped/4 -> Matrix Concatenate4/1
  Selector4/1 -> Independent Suspension - Mapped/2
  Selector10/1 -> Independent Suspension - Mapped/7
  Selector9/1 -> Independent Suspension - Mapped/6
  Wheel  Adapter/3(z) -> Bus Creator4/3
  Solid Axle Suspension - Mapped/2 -> Matrix Concatenate6/2
  Wheel/1 -> Wheel  Adapter/1(Wheels)
  Selector5/1 -> Independent Suspension - Mapped/1
  Independent Suspension - Mapped/3 -> Matrix Concatenate5/1
  Selector8/1 -> Independent Suspension - Mapped/5
  Independent Suspension - Mapped/2 -> Matrix Concatenate6/1
  Independent Suspension - Mapped/6 -> Matrix Concatenate2/1
  Selector20/1 -> Solid Axle Suspension - Mapped/2
  Independent Suspension - Mapped/1 -> Terminator/1
  Bus Creator2/1 -> Bus Creator3/1  "Veh"
  Bus Selector/4 -> Selector7/1, Selector21/1  "<Fx>"
  Matrix Concatenate2/1 -> Bus Creator1/4  "Ang"
  Wheel  Adapter/2(WhlFy) -> Bus Creator4/2  "Fy"
  Bus Creator4/1 -> Bus Selector/1
  Selector17/1 -> Solid Axle Suspension - Mapped/6
  Selector2/1 -> Independent Suspension - Mapped/9
  Wheel  Adapter/5(M) -> Bus Creator4/5
  Matrix Concatenate/1 -> Bus Creator1/3  "ydot"
  Steering/1 -> Steering Adapter/1(Steer)
  Matrix Concatenate1/1 -> Bus Creator1/2  "xdot"
  Selector15/1 -> Matrix Concatenate/2
  Selector3/1 -> Solid Axle Suspension - Mapped/1
  Bus Selector1/2 -> Selector11/1, Selector18/1  "<V>"
  Vehicle Adapter/1(VehSusp) -> Bus Selector1/1
  Steering Adapter/1(StrgAng) -> Selector2/1
  Selector6/1 -> Independent Suspension - Mapped/3
  Bus Selector/6 -> Selector9/1, Selector17/1  "<M>"
  Wheel  Adapter/1(WhlFx) -> Bus Creator4/1  "Fx"
  Selector11/1 -> Independent Suspension - Mapped/8
  Wheel  Adapter/6(Re) -> Bus Creator4/6
  Matrix Concatenate6/1 -> Bus Creator2/1  "F"
  Bus Selector1/1 -> Selector10/1, Selector1/1  "<P>"
  Solid Axle Suspension - Mapped/6 -> Matrix Concatenate2/2
  Bus Selector/1 -> Selector3/1, Selector5/1  "<z>"
  Bus Selector/5 -> Selector8/1, Selector16/1  "<Fy>"
  Bus Creator1/1 -> Bus Creator3/2  "Whl"
  Bus Creator3/1 -> Suspension/1
  Bus Selector/2 -> Selector20/1, Selector4/1  "<Re>"
  Steer Rate Adapter/1(AngVel) -> Bus Creator1/6
  Independent Suspension - Mapped/5 -> Terminator2/1
  Solid Axle Suspension - Mapped/5 -> Terminator3/1
  Selector19/1 -> Selector14/1, Selector15/1
  Selector23/1 -> Selector12/1, Selector13/1
  Bus Selector2/1 -> Bus Creator1/5  "<z>"
  Wheel1/1 -> Bus Selector2/1

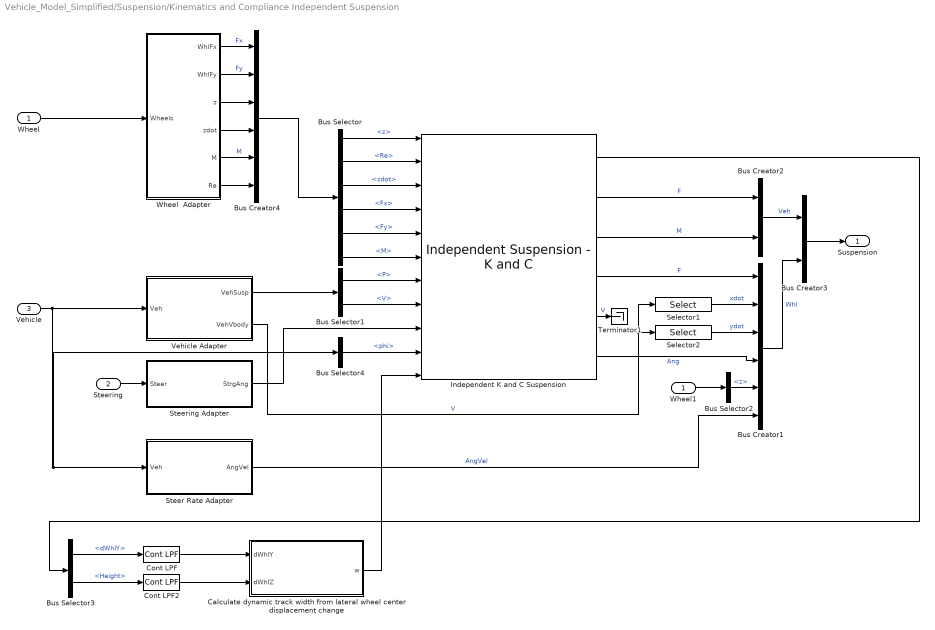
== system Vehicle_Model_Simplified/Suspension/Kinematics and Compliance Independent Suspension ==
  Wheel : Inport
  Steering : Inport  Port=2
  Vehicle : Inport  Port=3
  Bus Creator1 : BusCreator  Inputs=6
  Bus Creator2 : BusCreator  Inputs=2
  Bus Creator3 : BusCreator  Inputs=2
  Bus Creator4 : BusCreator  Inputs=6
  Bus Selector : BusSelector  OutputSignals=z,Re,zdot,Fx,Fy,M
  Bus Selector1 : BusSelector  OutputSignals=P,V
  Bus Selector2 : BusSelector  OutputSignals=SuspFrame.z
  Bus Selector3 : BusSelector  OutputSignals=dWhlY,Height
  Bus Selector4 : BusSelector  OutputSignals=InertFrm.Cg.Ang.phi
  Calculate dynamic track width from lateral wheel center displacement change : Subsystem  mask{w=VEH.TrackWidth.*[1 1]}
      mask prompts: w "vdynblks:vehdynVehBody6Dof:blkPrm_w"
      mask DialogControl w Prompt: Track widths [front, rear], w [m]:
  Cont LPF : autolibutils/Cont LPF  wc=100*2*pi  AbsoluteTolerance=auto  aMode=2
  Cont LPF2 : autolibutils/Cont LPF  wc=100*2*pi  AbsoluteTolerance=auto  aMode=2
  Independent K and C Suspension : vehdynlibsuspension/Independent Suspension - K and C  ActiveDampEn=off  NumAxl=2  NumWhlsByAxl=[2 2]  StrgEnByAxl=[1 0]  AntiSwayEnByAxl=[0 0]  WhlNumVec="[1  2  1  2]"  AxleNumVec="[1  1  2  2]"  SuspTypesByAxle="[1  1]"  SuspImage=suspkandc.png  IdealSuspEn=on  IdealSuspAxles="[1  2]"  tanTheta_FL=[0 0 0]  tanTheta_FR=[0 0 0]  tanTheta_RL=[0 0 0]  tanTheta_RR=[0 0 0]  SteerSign=1  LongitudinalSign=1  LateralSign=1  VerticalSign=1  WhlMzSign=1  tanTheta_SVSA_WC_FL=[0 0 0]  tanTheta_SVSA_WC_FR=[0 0 0]  tanTheta_SVSA_WC_RL=[0 0 0]  tanTheta_SVSA_WC_RR=[0 0 0]  tanTheta_SVSA_CP_FL=[0 0 0]  tanTheta_SVSA_CP_FR=[0 0 0]  tanTheta_SVSA_CP_RL=[0 0 0]  tanTheta_SVSA_CP_RR=[0 0 0]  SuspType=Independent front and rear  DrivetrainType=FWD  StrPlusDirection=Right  XPlusDirection=Front  YPlusDirection=Right  ZPlusDirection=Up  WhlMzDirection=Counter-clockwise  ShockType=Constant  ShckFrcVsCompRate=ShckFrcVsCompRate  MotRatios=MotRatios  BumpSteer=BumpSteer  BumpCamber=BumpCamber  BumpCaster=BumpCaster  LatWhlCtrDisp=LatWhlCtrDisp  LngWhlCtrDisp=LngWhlCtrDisp  NrmlWhlRates=NrmlWhlRates  NrmlWhlFrcOff=NrmlWhlFrcOff  RollSteer=[0 0 0 0]  RollCamber=[0 0 0 0]  RollCaster=[0 0 0 0]  RollStiffArb=RollStiffArb  RollStiffNoArb=RollStiffNoArb  RollStiffArbFrnt=800  RollStiffNoArbFrnt=0  RollStiffNoTwstRear=0  CambVsSteerAng=CambVsSteerAng  CastVsSteerAng=CastVsSteerAng  LngSteerCompl=LngSteerCompl  LngCambCompl=LngCambCompl  LngCastCompl=LngCastCompl  LngWhlCtrCompl=LngWhlCtrCompl  LatWhlCtrComplLngBrk=LatWhlCtrComplLngBrk  LatSteerCompl=LatSteerCompl  LatCambCompl=LatCambCompl  LatWhlCtrComplLat=LatWhlCtrComplLat  AlgnTrqSteerCompl=AlgnTrqSteerCompl  AlgnTrqCambCompl=AlgnTrqCambCompl  LatLdTrnsfr=struct('FL',[-2. -1.;0 0;2. 1.],'FR',[-2. 1.;0 0;2. -1.],'RL',[-2. -1.;0 0;2. 1.],'RR',[-2. 1.;0 0;2. -1.])  StatToe=StatToe  StatCamber=StatCamber  StatCaster=StatCaster  StatLdWhlR=StatLdWhlR  MappedSuspEn=off  RollParamEn=off
  Selector1 : Selector  NumberOfDimensions=2  IndexOptions=Index vector (dialog),Select all  Indices=1,1  OutputSizes=1,1
  Selector2 : Selector  NumberOfDimensions=2  IndexOptions=Index vector (dialog),Select all  Indices=2,1  OutputSizes=1,1
  Steer Rate Adapter : Subsystem
  Steering Adapter : Subsystem
  Terminator1 : Terminator
  Vehicle Adapter : Subsystem
  Wheel  Adapter : Subsystem
  Wheel1 : InportShadow
  Suspension : Outport  VectorParamsAs1DForOutWhenUnconnected=off
  wires:
  Bus Creator3/1 -> Suspension/1
  Bus Creator1/1 -> Bus Creator3/2  "Whl"
  Bus Selector1/2 -> Independent K and C Suspension/8  "<V>"
  Bus Selector/6 -> Independent K and C Suspension/6  "<M>"
  Bus Selector/5 -> Independent K and C Suspension/5  "<Fy>"
  Steering/1 -> Steering Adapter/1(Steer)
  Bus Selector/3 -> Independent K and C Suspension/3  "<zdot>"
  Bus Selector/4 -> Independent K and C Suspension/4  "<Fx>"
  Vehicle/1 -> Vehicle Adapter/1(Veh), Bus Selector4/1, Steer Rate Adapter/1(Veh)
  Vehicle Adapter/1(VehSusp) -> Bus Selector1/1
  Independent K and C Suspension/3 -> Bus Creator2/2  "M"
  Wheel  Adapter/2(WhlFy) -> Bus Creator4/2  "Fy"
  Wheel  Adapter/1(WhlFx) -> Bus Creator4/1  "Fx"
  Wheel/1 -> Wheel  Adapter/1(Wheels)
  Wheel  Adapter/3(z) -> Bus Creator4/3
  Wheel  Adapter/4(zdot) -> Bus Creator4/4
  Wheel  Adapter/5(M) -> Bus Creator4/5  "M"
  Wheel  Adapter/6(Re) -> Bus Creator4/6
  Bus Selector/2 -> Independent K and C Suspension/2  "<Re>"
  Selector1/1 -> Bus Creator1/2  "xdot"
  Selector2/1 -> Bus Creator1/3  "ydot"
  Bus Selector1/1 -> Independent K and C Suspension/7  "<P>"
  Bus Selector/1 -> Independent K and C Suspension/1  "<z>"
  Independent K and C Suspension/4 -> Bus Creator1/1  "F"
  Independent K and C Suspension/6 -> Bus Creator1/4  "Ang"
  Vehicle Adapter/2(VehVbody) -> Selector1/1, Selector2/1  "V"
  Independent K and C Suspension/2 -> Bus Creator2/1  "F"
  Bus Creator2/1 -> Bus Creator3/1  "Veh"
  Bus Creator4/1 -> Bus Selector/1
  Steer Rate Adapter/1(AngVel) -> Bus Creator1/6  "AngVel"
  Steering Adapter/1(StrgAng) -> Independent K and C Suspension/9
  Independent K and C Suspension/1 -> Bus Selector3/1
  Independent K and C Suspension/5 -> Terminator1/1  "V"
  Bus Selector2/1 -> Bus Creator1/5  "<z>"
  Wheel1/1 -> Bus Selector2/1
  Bus Selector4/1 -> Independent K and C Suspension/10  "<phi>"
  Calculate dynamic track width from lateral wheel center displacement change/1(w) -> Independent K and C Suspension/11
  Bus Selector3/1 -> Cont LPF/1  "<dWhlY>"
  Bus Selector3/2 -> Cont LPF2/1  "<Height>"
  Cont LPF/1 -> Calculate dynamic track width from lateral wheel center displacement change/1(dWhlY)
  Cont LPF2/1 -> Calculate dynamic track width from lateral wheel center displacement change/2(dWhlZ)
